simulink model "gtcs_math_v1_backup"  (R2022b)
settings: Solver=VariableStepAuto  StartTime=0.0  StopTime=10  RelTol=1e-3
undefined symbols (not defined in the file or in its folder): B_load, B_motor, B_reducer, GearRatio, J_load, J_motor, J_reducer, ke, kt, L_motor, R_motor, sigbuilder_block
libraries: slpidlib x2, simulink x2
settings Model: DataDictionary=gtcs_math_v1.sldd  Creator=yusuf.ogut  LastModifiedBy=Yusuf
settings ModelReferenceCC: EnableRefExpFcnMdlSchedulingChecks=on

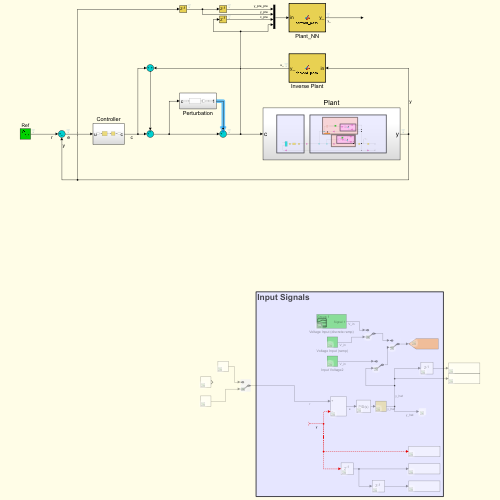
[thumbnail: Simulink's stored preview of the top-level diagram]
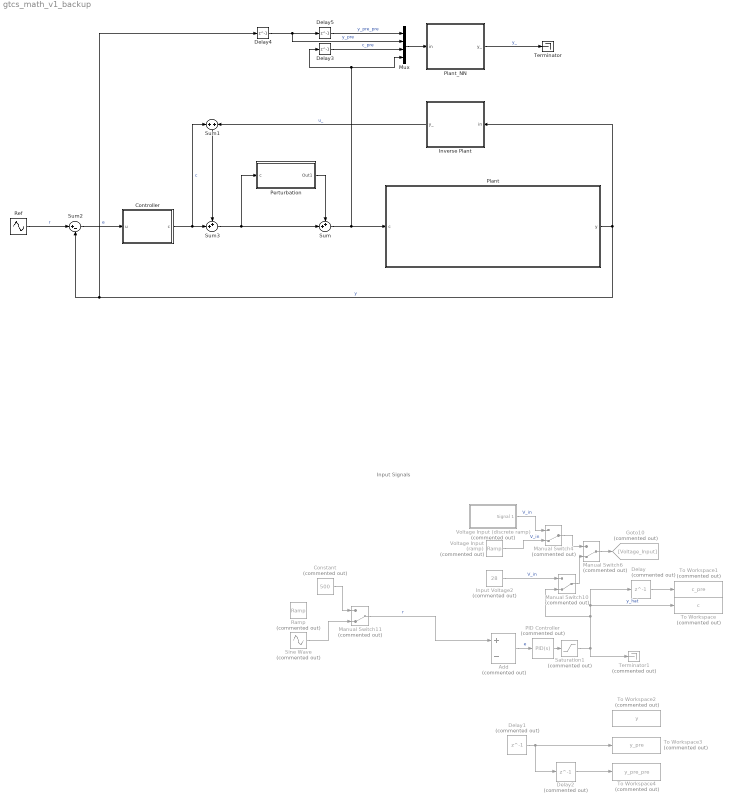
== system gtcs_math_v1_backup ==
  note: Input Signals
  Add : Sum  Commented=on  Inputs=+-
  Constant : Constant  Commented=on  Value=500
  Controller : Subsystem
  Delay : Delay  Commented=on  DelayLength=1  SampleTime=0.01
  Delay1 : Delay  Commented=on  DelayLength=1  SampleTime=0.01
  Delay2 : Delay  Commented=on  DelayLength=1  SampleTime=0.01
  Delay3 : Delay  DelayLength=1  SampleTime=0.01
  Delay4 : Delay  DelayLength=1  SampleTime=0.01
  Delay5 : Delay  DelayLength=1  SampleTime=0.01
  Goto10 : Goto  Commented=on  GotoTag=Voltage_Input
  Input Voltage2 : Constant  Commented=on  Value=28
  Inverse Plant : MATLAB Function  TreatAsAtomicUnit=on
  Manual Switch{4,6,10..11} (4 alike) : ManualSwitch  Commented=on  CurrentSetting=0
  Mux : Mux
  PID Controller : slpidlib/PID Controller  Commented=on  Controller=PID  Form=Parallel  TimeDomain=Continuous-time  UseExternalTs=off  SampleTime=-1  IntegratorMethod=Forward Euler  FilterMethod=Forward Euler  ControllerParametersSource=internal  P=1  I=0.12  UseKiTs=off  D=0  N=100  UseFilter=on  TunerSelectOption=Transfer Function Based (PID Tuner App)  InitialConditionSource=internal  InitialConditionForIntegrator=0  InitialConditionForFilter=0  DifferentiatorICPrevScaledInput=0  ExternalReset=none  TrackingMode=off  Kt=1  LimitOutput=off  SatLimitsSource=internal  UpperSaturationLimit=inf  LowerSaturationLimit=-inf  LinearizeAsGain=on  AntiWindupMode=none  Kb=1  LimitIntegrator=off  UpperIntegratorSaturationLimit=inf  LowerIntegratorSaturationLimit=-inf  POutMin=[]  POutMax=[]  IOutMin=[]  IOutMax=[]  DOutMin=[]  DOutMax=[]  NOutMin=[]  NOutMax=[]  SumOutMin=[]  SumOutMax=[]  SaturationOutMin=[]  SaturationOutMax=[]  PParamMin=[]  PParamMax=[]  IParamMin=[]  IParamMax=[]  DParamMin=[]  DParamMax=[]  NParamMin=[]  NParamMax=[]  KbParamMin=[]  KbParamMax=[]  KtParamMin=[]  KtParamMax=[]  KbOutMin=[]  KbOutMax=[]  KtOutMin=[]  KtOutMax=[]  IntegratorOutMin=[]  IntegratorOutMax=[]  FilterOutMin=[]  FilterOutMax=[]  SumI1OutMin=[]  SumI1OutMax=[]  SumI2OutMin=[]  SumI2OutMax=[]  SumI3OutMin=[]  SumI3OutMax=[]  SumI4OutMin=[]  SumI4OutMax=[]  SumDOutMin=[]  SumDOutMax=[]  DifferentiatorOutMin=[]  DifferentiatorOutMax=[]  FilterDiffOutCoefMin=[]  FilterDiffOutCoefMax=[]  ReciprocalOutMin=[]  ReciprocalOutMax=[]  SumDenOutMin=[]  SumDenOutMax=[]  SumNumOutMin=[]  SumNumOutMax=[]  DivideOutMin=[]  DivideOutMax=[]  UdiffTsProdOutMin=[]  UdiffTsProdOutMax=[]  NTsProdOutMin=[]  NTsProdOutMax=[]  UintegralTsProdOutMin=[]  UintegralTsProdOutMax=[]  UngainTsProdOutMin=[]  UngainTsProdOutMax=[]  ClampingZeroOutDataTypeStr=Inherit: Inherit via back propagation  ClampingZeroOutMin=[]  ClampingZeroOutMax=[]  FilterDenConstantOutDataTypeStr=Inherit: Inherit via back propagation  FilterDenConstantOutMin=[]  FilterDenConstantOutMax=[]  PCopyOutDataTypeStr=Inherit: Inherit via back propagation  PCopyOutMin=[]  PCopyOutMax=[]  NCopyOutDataTypeStr=Inherit: Inherit via back propagation  NCopyOutMin=[]  NCopyOutMax=[]  IntegratorContinuousStateAttributes=''  IntegratorStateMustResolveToSignalObject=off  IntegratorRTWStateStorageClass=Auto  FilterContinuousStateAttributes=''  FilterStateMustResolveToSignalObject=off  FilterRTWStateStorageClass=Auto  ParallelPVariant=InternalParameters  IdealPVariant=Disabled  IVariant=InternalParameters  DVariant=InternalParameters  IntegratorVariant=Continuous  SatVariant=Disabled  AWVariant=Passthrough  PCopyVariant=Disabled  TRVariant=Disabled  FdbkBlocksVariant=Forward  IdealPFdbkVariant=Disabled  SatFdbkVariant=Disabled  DerivativeFilterVariant=ContFilter  NVariant=InternalParameters  NCopyVariant=Disabled  FilterICVariant=InternalICsFilter  IntegratorICVariant=InternalICs  ExternalResetVariant=Disabled  TRSumVariant=Passthrough  SumFdbkVariant=Disabled  SumVariant=Sum_PID  TsampFilterVariant=InternalTs  TsampNgainVariant=Passthrough  TsampIntegralVariant=Passthrough  ExternalSaturationOutDataTypeStr=Inherit: Same as second input
  Perturbation : Subsystem
  Plant : Subsystem
  Plant_NN : MATLAB Function  TreatAsAtomicUnit=on
  Ramp : simulink/Sources/Ramp  Commented=on  slope=25  start=0  InitialOutput=0
  Ref : Sin  Amplitude=400  SampleTime=0
  Saturation1 : Saturate  Commented=on  UpperLimit=28  LowerLimit=-28
  Sine Wave : Sin  Commented=on  Amplitude=400  SampleTime=0
  Sum : Sum  Inputs=++|
  Sum1 : Sum  Inputs=+|+
  Sum2 : Sum  Inputs=|+-
  Sum3 : Sum  Inputs=++|
  Terminator : Terminator
  Terminator1 : Terminator  Commented=on
  To Workspace : ToWorkspace  Commented=on  VariableName=c  SampleTime=0.01
  To Workspace1 : ToWorkspace  Commented=on  VariableName=c_pre  SampleTime=0.01
  To Workspace2 : ToWorkspace  Commented=on  VariableName=y  SampleTime=0.01
  To Workspace3 : ToWorkspace  Commented=on  VariableName=y_pre  SampleTime=0.01
  To Workspace4 : ToWorkspace  Commented=on  VariableName=y_pre_pre  SampleTime=0.01
  Voltage Input (discrete ramp) : Subsystem  Tag=STV Subsys  Commented=on  LoadFcn=sigbuilder_block('load');  StartFcn=sigbuilder_block('start');  StopFcn=sigbuilder_block('stop');  ClipboardFcn=sigbuilder_block('clipboard');  mask(Sigbuilder block){tuvar=[0:10]}
      mask help: Simulink:masks:SigbuilderBlock_MD
      mask init:
      | if ~strcmp(get_param(bdroot(gcbh),'SimulationStatus'),'stopped') tuvar = sigbuilder_block('maskInit'); end
      settings: CopyFcn=sigbuilder_block('copy');  DeleteFcn=sigbuilder_block('delete');  ModelCloseFcn=sigbuilder_block('modelClose');  PreSaveFcn=sigbuilder_block('preSave');  PauseFcn=sigbuilder_block('pause');  ContinueFcn=sigbuilder_block('continue');  NameChangeFcn=sigbuilder_block('namechange');  OpenFcn=sigbuilder_block('open',[0.75 36.75 718.5 709.5 ]);  CloseFcn=sigbuilder_block('close');
      mask Display: plot(0, 0, 100, 100,[2, 2, 32, 32, 2], [68, 8, 8, 68, 68],[32, 2], [38, 38], [32, 19, 2],[53, 60, 44], [32, 17, 17, 2],[16, 16, 31, 31]);txt = getActiveGroup(gcbh);text(2, 100, txt,'verticalAlignment', 'top');
  Voltage Input (ramp) : simulink/Sources/Ramp  Commented=on  slope=0.5  start=50  InitialOutput=5
  wires:
  Voltage Input (discrete ramp)/1(Signal 1) -> Manual Switch4/1  "V_in"
  Voltage Input (ramp)/1 -> Manual Switch4/2  "V_in"
  Input Voltage2/1 -> Manual Switch10/1  "V_in"
  Manual Switch4/1 -> Manual Switch6/1
  Manual Switch6/1 -> Goto10/1
  ? -> To Workspace2/1, Delay1/1, Add/2  "y"
  Add/1 -> PID Controller/1  "e"
  PID Controller/1 -> Saturation1/1
  Manual Switch10/1 -> Manual Switch6/2
  Sine Wave/1 -> Manual Switch11/2
  Manual Switch11/1 -> Add/1  "r"
  Saturation1/1 -> Terminator1/1, Delay/1, To Workspace/1, Manual Switch10/2  "y_hat"
  Delay/1 -> To Workspace1/1
  Delay1/1 -> Delay2/1, To Workspace3/1
  Delay2/1 -> To Workspace4/1
  Constant/1 -> Manual Switch11/1
  Ref/1 -> Sum2/1  "r"
  Plant/1(y) -> Inverse Plant/1(in), Delay4/1, Sum2/2  "y"
  Sum2/1 -> Controller/1(u)  "e"
  Controller/1(c) -> Sum3/2, Sum1/1  "c"
  Plant_NN/1(y_) -> Terminator/1  "y_"
  Delay3/1 -> Mux/3  "c_pre"
  Delay4/1 -> Delay5/1, Mux/2  "y_pre"
  Delay5/1 -> Mux/1  "y_pre_pre"
  Mux/1 -> Plant_NN/1(in)
  Perturbation/1(Out1) -> Sum/1
  Sum/1 -> Plant/1(c), Mux/4, Delay3/1
  Sum1/1 -> Sum3/1
  Sum3/1 -> Perturbation/1(c), Sum/2
  Inverse Plant/1(y_) -> Sum1/2  "u_"

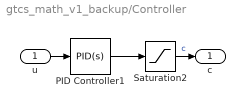
== system gtcs_math_v1_backup/Controller ==
  u : Inport
  PID Controller1 : slpidlib/PID Controller  Controller=PID  Form=Parallel  TimeDomain=Continuous-time  UseExternalTs=off  SampleTime=-1  IntegratorMethod=Forward Euler  FilterMethod=Forward Euler  ControllerParametersSource=internal  P=1  I=0.12  UseKiTs=off  D=0  N=100  UseFilter=on  TunerSelectOption=Transfer Function Based (PID Tuner App)  InitialConditionSource=internal  InitialConditionForIntegrator=0  InitialConditionForFilter=0  DifferentiatorICPrevScaledInput=0  ExternalReset=none  TrackingMode=off  Kt=1  LimitOutput=off  SatLimitsSource=internal  UpperSaturationLimit=inf  LowerSaturationLimit=-inf  LinearizeAsGain=on  AntiWindupMode=none  Kb=1  LimitIntegrator=off  UpperIntegratorSaturationLimit=inf  LowerIntegratorSaturationLimit=-inf  POutMin=[]  POutMax=[]  IOutMin=[]  IOutMax=[]  DOutMin=[]  DOutMax=[]  NOutMin=[]  NOutMax=[]  SumOutMin=[]  SumOutMax=[]  SaturationOutMin=[]  SaturationOutMax=[]  PParamMin=[]  PParamMax=[]  IParamMin=[]  IParamMax=[]  DParamMin=[]  DParamMax=[]  NParamMin=[]  NParamMax=[]  KbParamMin=[]  KbParamMax=[]  KtParamMin=[]  KtParamMax=[]  KbOutMin=[]  KbOutMax=[]  KtOutMin=[]  KtOutMax=[]  IntegratorOutMin=[]  IntegratorOutMax=[]  FilterOutMin=[]  FilterOutMax=[]  SumI1OutMin=[]  SumI1OutMax=[]  SumI2OutMin=[]  SumI2OutMax=[]  SumI3OutMin=[]  SumI3OutMax=[]  SumI4OutMin=[]  SumI4OutMax=[]  SumDOutMin=[]  SumDOutMax=[]  DifferentiatorOutMin=[]  DifferentiatorOutMax=[]  FilterDiffOutCoefMin=[]  FilterDiffOutCoefMax=[]  ReciprocalOutMin=[]  ReciprocalOutMax=[]  SumDenOutMin=[]  SumDenOutMax=[]  SumNumOutMin=[]  SumNumOutMax=[]  DivideOutMin=[]  DivideOutMax=[]  UdiffTsProdOutMin=[]  UdiffTsProdOutMax=[]  NTsProdOutMin=[]  NTsProdOutMax=[]  UintegralTsProdOutMin=[]  UintegralTsProdOutMax=[]  UngainTsProdOutMin=[]  UngainTsProdOutMax=[]  ClampingZeroOutDataTypeStr=Inherit: Inherit via back propagation  ClampingZeroOutMin=[]  ClampingZeroOutMax=[]  FilterDenConstantOutDataTypeStr=Inherit: Inherit via back propagation  FilterDenConstantOutMin=[]  FilterDenConstantOutMax=[]  PCopyOutDataTypeStr=Inherit: Inherit via back propagation  PCopyOutMin=[]  PCopyOutMax=[]  NCopyOutDataTypeStr=Inherit: Inherit via back propagation  NCopyOutMin=[]  NCopyOutMax=[]  IntegratorContinuousStateAttributes=''  IntegratorStateMustResolveToSignalObject=off  IntegratorRTWStateStorageClass=Auto  FilterContinuousStateAttributes=''  FilterStateMustResolveToSignalObject=off  FilterRTWStateStorageClass=Auto  ParallelPVariant=InternalParameters  IdealPVariant=Disabled  IVariant=InternalParameters  DVariant=InternalParameters  IntegratorVariant=Continuous  SatVariant=Disabled  AWVariant=Passthrough  PCopyVariant=Disabled  TRVariant=Disabled  FdbkBlocksVariant=Forward  IdealPFdbkVariant=Disabled  SatFdbkVariant=Disabled  DerivativeFilterVariant=ContFilter  NVariant=InternalParameters  NCopyVariant=Disabled  FilterICVariant=InternalICsFilter  IntegratorICVariant=InternalICs  ExternalResetVariant=Disabled  TRSumVariant=Passthrough  SumFdbkVariant=Disabled  SumVariant=Sum_PID  TsampFilterVariant=InternalTs  TsampNgainVariant=Passthrough  TsampIntegralVariant=Passthrough  ExternalSaturationOutDataTypeStr=Inherit: Same as second input
  Saturation2 : Saturate  UpperLimit=28  LowerLimit=-28
  c : Outport
  wires:
  Saturation2/1 -> c/1  "c"
  PID Controller1/1 -> Saturation2/1
  u/1 -> PID Controller1/1

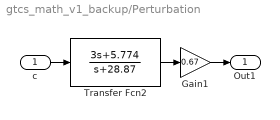
== system gtcs_math_v1_backup/Perturbation ==
  c : Inport
  Gain1 : Gain  Gain=0.67
  Transfer Fcn2 : TransferFcn  Numerator=[3 5.774]  Denominator=[1 28.87]
  Out1 : Outport
  wires:
  c/1 -> Transfer Fcn2/1
  Transfer Fcn2/1 -> Gain1/1
  Gain1/1 -> Out1/1

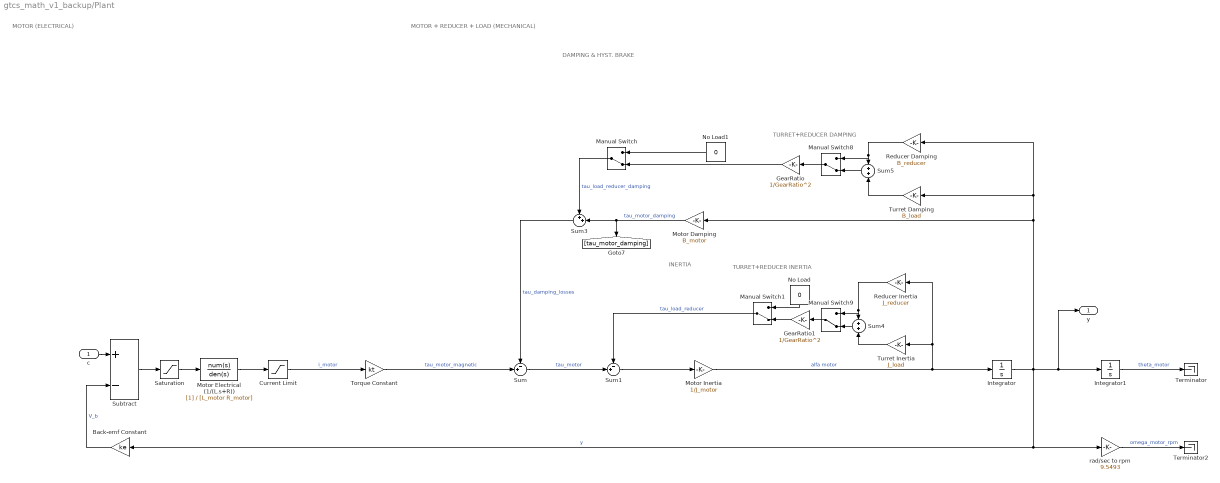
== system gtcs_math_v1_backup/Plant ==
  note: TURRET+REDUCER INERTIA
  note: TURRET+REDUCER DAMPING
  note: DAMPING & HYST. BRAKE
  note: INERTIA
  note: MOTOR (ELECTRICAL)
  note: MOTOR + REDUCER + LOAD (MECHANICAL)
  c : Inport
  Back-emf Constant : Gain  Gain=ke
  Current Limit : Saturate  UpperLimit=80  LowerLimit=-80
  GearRatio : Gain  Gain=1/GearRatio^2
  GearRatio1 : Gain  Gain=1/GearRatio^2
  Integrator : Integrator
  Integrator1 : Integrator
  Manual Switch{,1,8..9} (4 alike) : ManualSwitch  CurrentSetting=0
  Motor Damping : Gain  Gain=B_motor
  Motor Electrical (1/(L.s+R)) : TransferFcn  Denominator=[L_motor R_motor]
  Motor Inertia : Gain  Gain=1/J_motor
  No Load : Constant  Value=0
  No Load1 : Constant  Value=0
  Reducer Damping : Gain  Gain=B_reducer
  Reducer Inertia : Gain  Gain=J_reducer
  Saturation : Saturate  UpperLimit=28  LowerLimit=-28
  Subtract : Sum  Inputs=+-
  Sum : Sum  Inputs=-+|
  Sum1 : Sum  Inputs=-+|
  Sum3 : Sum  Inputs=++|
  Sum4 : Sum
  Sum5 : Sum
  Terminator : Terminator
  Terminator2 : Terminator
  Torque Constant : Gain  Gain=kt
  Turret Damping : Gain  Gain=B_load
  Turret Inertia : Gain  Gain=J_load
  rad/sec to rpm : Gain  Gain=9.5493
  y : Outport
  wires:
  No Load/1 -> Manual Switch1/1
  Turret Damping/1 -> Sum5/2
  Reducer Inertia/1 -> Manual Switch9/1, Sum4/1
  GearRatio1/1 -> Manual Switch1/2
  Torque Constant/1 -> Sum/2  "tau_motor_magnetic"
  Manual Switch/1 -> Sum3/1  "tau_load_reducer_damping"
  Integrator/1 -> y/1, Integrator1/1, rad/sec to rpm/1, Back-emf Constant/1, Turret Damping/1, Reducer Damping/1, Motor Damping/1  "y"
  Current Limit/1 -> Torque Constant/1  "i_motor"
  No Load1/1 -> Manual Switch/1
  Manual Switch9/1 -> GearRatio1/1
  Sum3/1 -> Sum/1  "tau_damping_losses"
  Motor Inertia/1 -> Integrator/1, Turret Inertia/1, Reducer Inertia/1  "alfa motor"
  Sum4/1 -> Manual Switch9/2
  Sum1/1 -> Motor Inertia/1
  Manual Switch1/1 -> Sum1/1  "tau_load_reducer"
  GearRatio/1 -> Manual Switch/2
  Integrator1/1 -> Terminator/1  "theta_motor"
  Turret Inertia/1 -> Sum4/2
  Manual Switch8/1 -> GearRatio/1
  Reducer Damping/1 -> Manual Switch8/1, Sum5/1
  Sum/1 -> Sum1/2  "tau_motor"
  Motor Damping/1 -> [tau_motor_damping], Sum3/2  "tau_motor_damping"
  Sum5/1 -> Manual Switch8/2
  Saturation/1 -> Motor Electrical (1/(L.s+R))/1
  Back-emf Constant/1 -> Subtract/2  "V_b"
  c/1 -> Subtract/1
  rad/sec to rpm/1 -> Terminator2/1  "omega_motor_rpm"
  Motor Electrical (1/(L.s+R))/1 -> Current Limit/1
  Subtract/1 -> Saturation/1

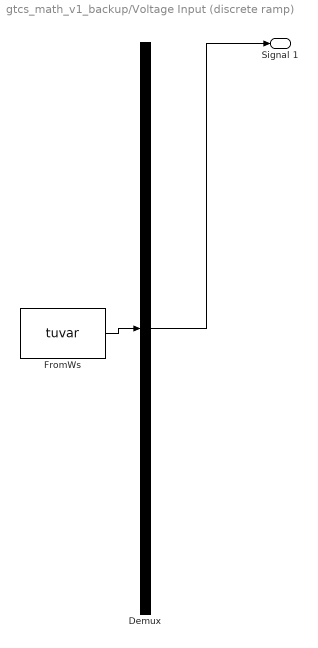
== system gtcs_math_v1_backup/Voltage Input (discrete ramp) ==
  Demux : Demux  Tag=STV Demux  Outputs=1
      settings: DisplayOption=none
  FromWs : FromWorkspace  Tag=STV FromWs  VariableName=tuvar
      SigBuilderData=|
      | common.afterFinalStr = 'Extrapolate'
      | common.sampleTime = 0
      | dataSet.timeRange = [0 34]
      | dataSet.name = 'Group 1'
      | sbobj.Groups.Name = 'Group 1'
      | sbobj.Groups.Signals.Name = 'Signal 1'
      | sbobj.Groups.Signals.XData = [0 8 10 12 14 16 18 20 22 24 26 28 30 32 34]
      | sbobj.Groups.Signals.YData = [0 3.27 3.27 7.28 7.28 11.23 11.23 15.19 15.19 19.17 19.17 23.18 23.18 32 32]
      | sbobj.Groups.TimeRange = [0 34]
  Signal 1 : Outport  Tag=STV Outport
  wires:
  FromWs/1 -> Demux/1
  Demux/1 -> Signal 1/1

== matlab function gtcs_math_v1_backup/Inverse Plant ==
  data: in input; y_ output
function y_ = forward_pass(in)
    c_ =  0.0534; r_ = 16.0258;
    c__ = 1.2811; r__ = 384.4721;
    input_training = (in - c__)/r__;
    Phi = [ -0.7229   -0.1132         0         0
            -0.7229   -0.1132         0         0
            -0.7229   -0.1132         0         0
            -0.4882   -0.4882   -0.4882   -0.1223];
    BIAS = -.1;
    % FORWARD PASS:
    NUM_INP = 1; NUM_HID = 3;
    input_vector = [input_training;BIAS];
    S1 = Phi(1:NUM_HID,1:NUM_INP+1)*input_vector;
    O1 = tanh(S1);
    S2 = Phi(NUM_HID+1:end,1:NUM_HID+1)*[O1;BIAS];
    y_ = S2*r_+c_;
end

== matlab function gtcs_math_v1_backup/Plant_NN ==
  data: in input; y_ output
function y_ = forward_pass(in)
    c_sf_i_4 = 24.3519;     r_sf_i_4 = 3.6481;
    c_sf_i_3 = 14;          r_sf_i_3 = 14;
    c_sf_i_2 = 249.4384;    r_sf_i_2 = 249.4384;
    c_sf_i_1 = 249.4394;    r_sf_i_1 = 249.4394;
    c_sf_o_1 = 249.3494;    r_sf_o_1 = 249.4394;
    input_training = (([in(4) in(3) in(2) in(1)] - [c_sf_i_4 c_sf_i_3 c_sf_i_2 c_sf_i_1]) ./ [r_sf_i_4 r_sf_i_3 r_sf_i_2 r_sf_i_1])';

    Phi = [     0.0386   -0.0713   -0.3476   -0.3525    0.0122         0         0         0         0         0         0
                0.0386   -0.0713   -0.3476   -0.3525    0.0122         0         0         0         0         0         0
                0.0386   -0.0713   -0.3476   -0.3525    0.0122         0         0         0         0         0         0
                0.0386   -0.0713   -0.3476   -0.3525    0.0122         0         0         0         0         0         0
                0.0386   -0.0713   -0.3476   -0.3525    0.0122         0         0         0         0         0         0
                0.0386   -0.0713   -0.3476   -0.3525    0.0122         0         0         0         0         0         0
                0.0386   -0.0713   -0.3476   -0.3525    0.0122         0         0         0         0         0         0
                0.0386   -0.0713   -0.3476   -0.3525    0.0122         0         0         0         0         0         0
                0.0386   -0.0713   -0.3476   -0.3525    0.0122         0         0         0         0         0         0
                0.0386   -0.0713   -0.3476   -0.3525    0.0122         0         0         0         0         0         0
               -0.1525   -0.1525   -0.1525   -0.1525   -0.1525   -0.1525   -0.1525   -0.1525   -0.1525   -0.1525   -0.1037];
    BIAS = -.1;
    % FORWARD PASS:
    NUM_INP = 4; NUM_HID = 10;
    input_vector = [input_training;BIAS];
    S1 = Phi(1:NUM_HID,1:NUM_INP+1)*input_vector;
    O1 = tanh(S1);
    S2 = Phi(NUM_HID+1:end,1:NUM_HID+1)*[O1;BIAS];
    y_ = S2 * r_sf_o_1 + c_sf_o_1;
end
